simulink model "softarm_tendon_actuation_demo"  (R2025a)
settings: Solver=ode15s  StartTime=0.0  StopTime=0.5  RelTol=1e-3
PreLoadFcn:
  | softarm_model_dir=fileparts(get_param(bdroot,'FileName'));softarm_root=fileparts(fileparts(softarm_model_dir));addpath(fullfile(softarm_root,'matlab'));addpath(fullfile(softarm_root,'matlab','simulink'));
InitFcn:
  | softarm_model_dir=fileparts(get_param(bdroot,'FileName'));softarm_root=fileparts(fileparts(softarm_model_dir));addpath(fullfile(softarm_root,'matlab'));addpath(fullfile(softarm_root,'matlab','simulink'));softarm_plant_block=string(bdroot)+"/Plant";softarm_actuator_block=string(bdroot)+"/Actuator mode";softarm_mode=string(get_param(softarm_actuator_block,'Mode'));set_param(softarm_actuator_block,'LabelModeActiveChoice',char(softarm_mode));if softarm_mode=="Acceleration",softarm_requirement="strict";else,softarm_requirement="force";end;softarm.applyPlantMask(softarm_plant_block,softarm_requirement);
undefined symbols (not defined in the file): softarm_narm, softarm_nq, softarm_u0, softarm_x0
settings Model: Creator=rlwan  LastModifiedBy=rlwan
settings DataIOCC: ReturnWorkspaceOutputs=off

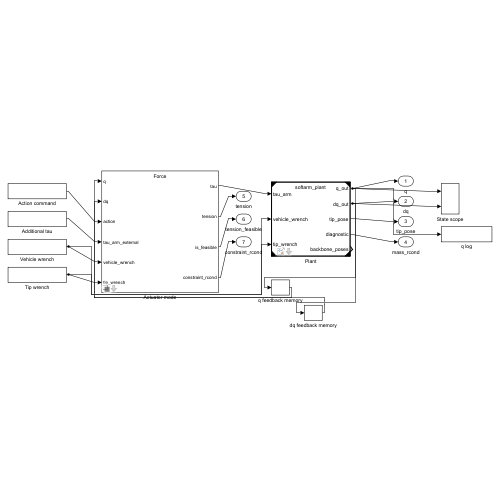
[thumbnail: Simulink's stored preview of the top-level diagram]
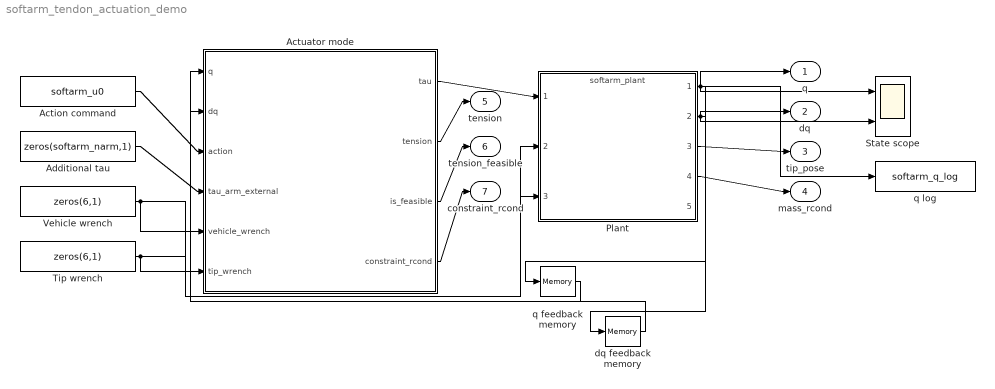
== system softarm_tendon_actuation_demo ==
  Action command : Constant  Value=softarm_u0
  Actuator mode : Subsystem  Variant=on  VariantControlMode=label  LabelModeActiveChoice=Force  mask{Mode=Force}
      mask prompts: Mode "Actuation mode"
      mask help: Select tendon tension or strict tendon-coordinate acceleration actuation.
      mask TypeOptions Mode: Force | Acceleration
      mask Callback Mode: softarm_mode=string(get_param(gcb,'Mode'));set_param(gcb,'LabelModeActiveChoice',char(softarm_mode));if softarm_mode=="Acceleration",softarm_requirement="strict";else,softarm_requirement="force";end;softarm.applyPlantMask(string(bdroot(gcb))+"/Plant",softarm_requirement);
  Additional tau : Constant  Value=zeros(softarm_narm,1)
  Plant : ModelReference  ModelNameDialog=softarm_plant  ParameterArgumentNames=Bundle  ParameterArgumentValues=Bundle  UsingDefaultArgumentValue=0  ModelReferenceVersion=1.1  Bundle='../generated/extensible_euler_bernoulli_pcs_three_tendon_n2'
  State scope : Scope  NumInputPorts=2
  Tip wrench : Constant  Value=zeros(6,1)
  Vehicle wrench : Constant  Value=zeros(6,1)
  dq feedback memory : Memory  InitialCondition=zeros(softarm_nq,1)
  q feedback memory : Memory  InitialCondition=softarm_x0(1:softarm_nq)
  q log : ToWorkspace  VariableName=softarm_q_log  SaveFormat=Timeseries  SampleTime=-1
  q : Outport
  dq : Outport  Port=2
  tip_pose : Outport  Port=3
  mass_rcond : Outport  Port=4
  tension : Outport  Port=5
  tension_feasible : Outport  Port=6
  constraint_rcond : Outport  Port=7
  wires:
  Plant/1 -> q log/1, q feedback memory/1, q/1, State scope/1
  q feedback memory/1 -> Actuator mode/1(q)
  Plant/2 -> dq feedback memory/1, dq/1, State scope/2
  dq feedback memory/1 -> Actuator mode/2(dq)
  Action command/1 -> Actuator mode/3(action)
  Additional tau/1 -> Actuator mode/4(tau_arm_external)
  Vehicle wrench/1 -> Actuator mode/5(vehicle_wrench), Plant/2
  Tip wrench/1 -> Actuator mode/6(tip_wrench), Plant/3
  Actuator mode/1(tau) -> Plant/1
  Actuator mode/2(tension) -> tension/1
  Actuator mode/3(is_feasible) -> tension_feasible/1
  Actuator mode/4(constraint_rcond) -> constraint_rcond/1
  Plant/3 -> tip_pose/1
  Plant/4 -> mass_rcond/1

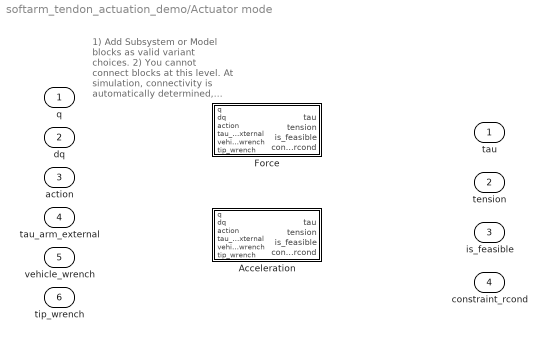
== system softarm_tendon_actuation_demo/Actuator mode ==
  note: 1) Add Subsystem or Model blocks as valid variant choices.
      | 2) You cannot connect blocks at this level. At simulation, connectivity is automatically
      | determined, based on the active variant and port name matching.
  q : Inport  PortDimensions=softarm_nq
  dq : Inport  Port=2  PortDimensions=softarm_nq
  action : Inport  Port=3  PortDimensions=softarm_nu
  tau_arm_external : Inport  Port=4  PortDimensions=softarm_narm
  vehicle_wrench : Inport  Port=5  PortDimensions=6
  tip_wrench : Inport  Port=6  PortDimensions=6
  Acceleration : Subsystem  VariantControl=Acceleration
  Force : Subsystem  VariantControl=Force
  tau : Outport
  tension : Outport  Port=2
  is_feasible : Outport  Port=3
  constraint_rcond : Outport  Port=4

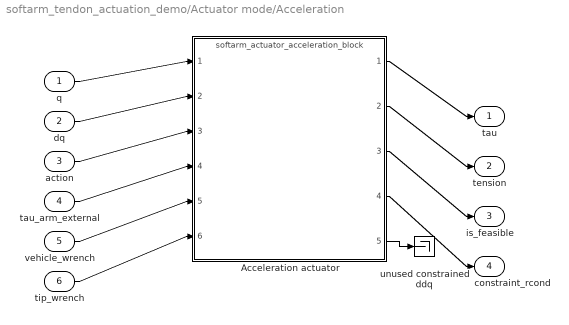
== system softarm_tendon_actuation_demo/Actuator mode/Acceleration ==
  q : Inport  PortDimensions=softarm_nq
  dq : Inport  Port=2  PortDimensions=softarm_nq
  action : Inport  Port=3  PortDimensions=softarm_nu
  tau_arm_external : Inport  Port=4  PortDimensions=softarm_narm
  vehicle_wrench : Inport  Port=5  PortDimensions=6
  tip_wrench : Inport  Port=6  PortDimensions=6
  Acceleration actuator : ModelReference  ModelNameDialog=softarm_actuator_acceleration_block  ModelReferenceVersion=1.1
  unused constrained ddq : Terminator
  tau : Outport
  tension : Outport  Port=2
  is_feasible : Outport  Port=3
  constraint_rcond : Outport  Port=4
  wires:
  q/1 -> Acceleration actuator/1
  dq/1 -> Acceleration actuator/2
  action/1 -> Acceleration actuator/3
  tau_arm_external/1 -> Acceleration actuator/4
  vehicle_wrench/1 -> Acceleration actuator/5
  tip_wrench/1 -> Acceleration actuator/6
  Acceleration actuator/1 -> tau/1
  Acceleration actuator/2 -> tension/1
  Acceleration actuator/3 -> is_feasible/1
  Acceleration actuator/4 -> constraint_rcond/1
  Acceleration actuator/5 -> unused constrained ddq/1

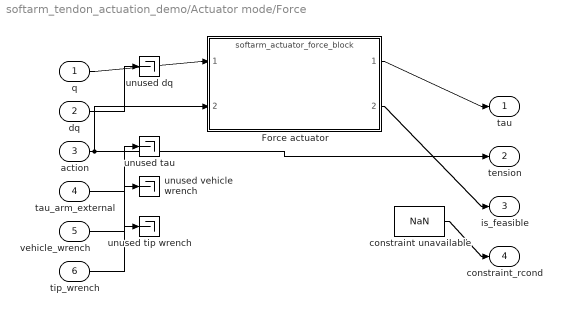
== system softarm_tendon_actuation_demo/Actuator mode/Force ==
  q : Inport  PortDimensions=softarm_nq
  dq : Inport  Port=2  PortDimensions=softarm_nq
  action : Inport  Port=3  PortDimensions=softarm_nu
  tau_arm_external : Inport  Port=4  PortDimensions=softarm_narm
  vehicle_wrench : Inport  Port=5  PortDimensions=6
  tip_wrench : Inport  Port=6  PortDimensions=6
  Force actuator : ModelReference  ModelNameDialog=softarm_actuator_force_block  ModelReferenceVersion=1.1
  constraint unavailable : Constant  Value=NaN
  unused dq : Terminator
  unused tau : Terminator
  unused tip wrench : Terminator
  unused vehicle wrench : Terminator
  tau : Outport
  tension : Outport  Port=2
  is_feasible : Outport  Port=3
  constraint_rcond : Outport  Port=4
  wires:
  q/1 -> Force actuator/1
  action/1 -> Force actuator/2, tension/1
  Force actuator/1 -> tau/1
  Force actuator/2 -> is_feasible/1
  constraint unavailable/1 -> constraint_rcond/1
  dq/1 -> unused dq/1
  tau_arm_external/1 -> unused tau/1
  vehicle_wrench/1 -> unused vehicle wrench/1
  tip_wrench/1 -> unused tip wrench/1
